simulink model "MCHP_SMO_MCLV48V300W_dsPIC33CK64MC105_DIM"  (R2022b)
settings: Solver=FixedStepDiscrete  StartTime=0.0  StopTime=10.0  FixedStep=50e-6  RelTol=1e-3  EnableMultiTasking=on
undefined symbols (not defined in the file): A4, B0, C12, C13, C4, C5, C6, C8, C9, DiscIntNeverNeededParam, inverter, Iq_Ref_openLoop, Max, MaxPer, ms, NumBits1, NumBits2, P20, P32, P52, P53, P54, P56, P57, P60, P61, PI_params, Pin, pmsm, PU_System, PWM1max, PWM_frequency, Resol, s, Speed_Ref_openLoop, Ts, Ts_speed, us
libraries: simulink x30, MCHP_Blockset x18, mcbcontrolslib x9, slpidlib x3, mcbplantlib x1, autolibpmsmexterior x1
(part 3 of 4)

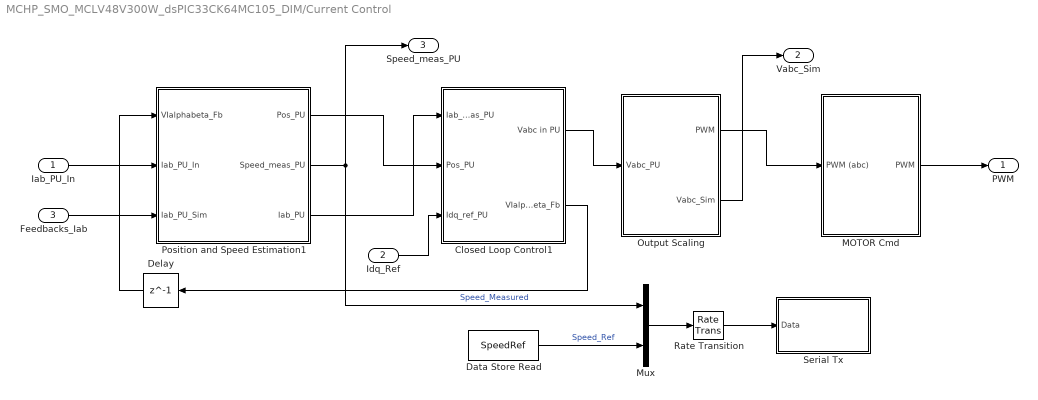
== system MCHP_SMO_MCLV48V300W_dsPIC33CK64MC105_DIM/Current Control ==
  Iab_PU_In : Inport
  Idq_Ref : Inport  Port=2
  Feedbacks_Iab : Inport  Port=3
  Closed Loop Control1 : Subsystem
  Data Store Read : DataStoreRead  DataStoreName=SpeedRef  IndexOptions=Index vector (dialog)  Indices=1  OutputSizes=1
  Delay : Delay  DelayLength=1
  MOTOR Cmd : Subsystem
  Mux : Mux  Inputs=2
  Output Scaling : Subsystem
  Position and Speed Estimation1 : Subsystem
  Rate Transition : RateTransition  Integrity=off  Deterministic=off  OutPortSampleTime=Ts*100
  Serial Tx : Subsystem
  PWM : Outport
  Vabc_Sim : Outport  Port=2
  Speed_meas_PU : Outport  Port=3
  wires:
  Output Scaling/1(PWM) -> MOTOR Cmd/1(PWM (abc))
  Closed Loop Control1/1(Vabc in PU) -> Output Scaling/1(Vabc_PU)
  MOTOR Cmd/1(PWM) -> PWM/1
  Iab_PU_In/1 -> Position and Speed Estimation1/2(Iab_PU_In)
  Closed Loop Control1/2(VIalphabeta_Fb) -> Delay/1
  Delay/1 -> Position and Speed Estimation1/1(VIalphabeta_Fb)
  Idq_Ref/1 -> Closed Loop Control1/3(Idq_ref_PU)
  Position and Speed Estimation1/1(Pos_PU) -> Closed Loop Control1/2(Pos_PU)
  Position and Speed Estimation1/3(Iab_PU) -> Closed Loop Control1/1(Iab_meas_PU)
  Feedbacks_Iab/1 -> Position and Speed Estimation1/3(Iab_PU_Sim)
  Output Scaling/2(Vabc_Sim) -> Vabc_Sim/1
  Data Store Read/1 -> Mux/2  "Speed_Ref"
  Rate Transition/1 -> Serial Tx/1(Data)
  Position and Speed Estimation1/2(Speed_meas_PU) -> Mux/1, Speed_meas_PU/1  "Speed_Measured"
  Mux/1 -> Rate Transition/1

== system MCHP_SMO_MCLV48V300W_dsPIC33CK64MC105_DIM/Inverter and Motor ==
  Duty_Cycles : Inport
  Codegeneration : Subsystem
  Simulation : Subsystem
  Variant Sink : VariantSink
  Variant Source : VariantSource
  Feedbacks_Iab : Outport  VectorParamsAs1DForOutWhenUnconnected=off
  wires:
  Codegeneration/1(Feedbacks_Iab) -> Variant Source/1
  Variant Sink/1 -> Codegeneration/1(Duty_Cycles)
  Simulation/1(Feedbacks_Iab) -> Variant Source/2
  Variant Sink/2 -> Simulation/1(Duty_Cycles)
  Variant Source/1 -> Feedbacks_Iab/1
  Duty_Cycles/1 -> Variant Sink/1

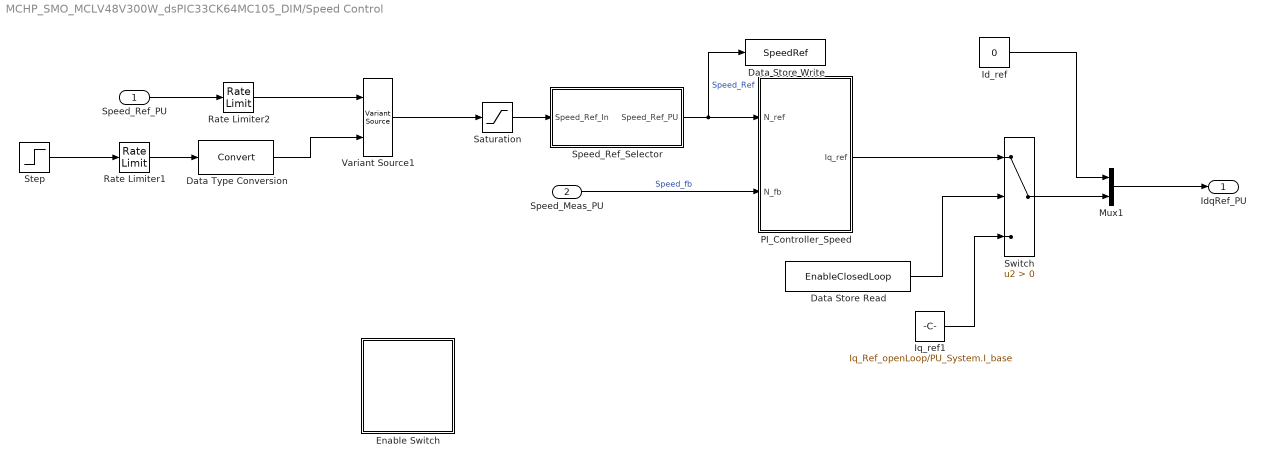
== system MCHP_SMO_MCLV48V300W_dsPIC33CK64MC105_DIM/Speed Control ==
  Speed_Ref_PU : Inport
  Speed_Meas_PU : Inport  Port=2
  Data Store Read : DataStoreRead  DataStoreName=EnableClosedLoop  IndexOptions=Index vector (dialog)  Indices=1  OutputSizes=1
  Data Store Write : DataStoreWrite  DataStoreName=SpeedRef  IndexOptions=Index vector (dialog)  Indices=1  OutputSizes=1
  Data Type Conversion : DataTypeConversion  SaturateOnIntegerOverflow=off  RndMeth=Floor
  Enable Switch : Subsystem  Variant=on  VariantControlMode=sim codegen switching
  Id_ref : Constant  Value=0  OutDataTypeStr=dataType  SampleTime=Ts_speed
  Iq_ref1 : Constant  Value=Iq_Ref_openLoop/PU_System.I_base  OutDataTypeStr=dataType  SampleTime=Ts_speed
  Mux1 : Mux  Inputs=2
  PI_Controller_Speed : Subsystem
  Rate Limiter1 : RateLimiter  RisingSlewLimit=0.5  FallingSlewLimit=-0.2  SampleTimeMode=inherited
  Rate Limiter2 : RateLimiter  RisingSlewLimit=0.5  FallingSlewLimit=-0.2  SampleTimeMode=inherited
  Saturation : Saturate  UpperLimit=(pmsm.N_max/PU_System.N_base)  LowerLimit=Speed_Ref_openLoop/PU_System.N_base
  Speed_Ref_Selector : Subsystem
  Step : Step  Time=5.5  Before=Speed_Ref_openLoop/PU_System.N_base
  Switch : Switch  Criteria=u2 > Threshold  SaturateOnIntegerOverflow=off  InputSameDT=off
  Variant Source1 : VariantSource
  IdqRef_PU : Outport  VectorParamsAs1DForOutWhenUnconnected=off
  wires:
  PI_Controller_Speed/1(Iq_ref) -> Switch/1
  Saturation/1 -> Speed_Ref_Selector/1(Speed_Ref_In)
  Data Store Read/1 -> Switch/2
  Iq_ref1/1 -> Switch/3
  Mux1/1 -> IdqRef_PU/1
  Speed_Ref_PU/1 -> Rate Limiter2/1
  Switch/1 -> Mux1/2
  Speed_Ref_Selector/1(Speed_Ref_PU) -> Data Store Write/1, PI_Controller_Speed/1(N_ref)  "Speed_Ref"
  Id_ref/1 -> Mux1/1
  Speed_Meas_PU/1 -> PI_Controller_Speed/2(N_fb)  "Speed_fb"
  Rate Limiter1/1 -> Data Type Conversion/1
  Data Type Conversion/1 -> Variant Source1/2
  Step/1 -> Rate Limiter1/1
  Rate Limiter2/1 -> Variant Source1/1
  Variant Source1/1 -> Saturation/1

== system MCHP_SMO_MCLV48V300W_dsPIC33CK64MC105_DIM/Triggered Subsystem ==
  Trigger : TriggerPort  TriggerType=falling  VariantControl=Variant
  Data Store Write : DataStoreWrite  DataStoreName=Enable  IndexOptions=Index vector (dialog)  Indices=1  OutputSizes=1
  Delay : Delay  DelayLength=1  InitialCondition=0
  NOT : Logic  Operator=NOT  IconShape=distinctive  AllPortsSameDT=off  OutDataTypeStr=boolean
  wires:
  NOT/1 -> Data Store Write/1, Delay/1
  Delay/1 -> NOT/1

== system MCHP_SMO_MCLV48V300W_dsPIC33CK64MC105_DIM/BOARD MCLV-48V-300W dsPIC33CK64MC105 MC DIM/ADC ==
  ADC dsPIC High Speed SAR Motor Currents : MCHP_Blockset/Analog IO/ADC dsPIC High Speed SAR  ACLKCON=Optimized for PWM resolution & ADC conversion speed  ADC_FRACT=Fractional (left aligned)  ADC_NRE=off  DMA_Size=Single trigger - (default)  ADC_Synchronisation=Triggered by custom source  ADC_Trig=Dynamic Options  ADC_Trig_TXT=PWM1 Trigger 1  ADC_TrigTimeStep=Trig model step after all sample from this block are converted  ADC_TrigInfo=0  SampleTime=50e-6  S_INPUT=[]  S_INPUT_Size=[]  S_OUTPUT="[5  5]"  S_OUTPUT_Size="[1  1]"  S_ListCustomDatatype=S.S_ListCustomDatatype={};  MCHP_USER_INTERRUPTS={ADCAN-1}{ADCBUF-1}{ADC Data -1 Ready}{VectorName(ADCAN-1Interrupt) Priority(-1) RegisterReadClear(ADCBUF-1)Config_BitSet(ADIELbits.IE-1) };{ADCAN0}{ADCBUF0}{ADC Data 0 Ready}{VectorName(ADCAN0Interrupt) Priority(-1) RegisterReadClear(ADCBUF0)Config_BitSet(ADIELbits.IE0) };  MCHP_PORT={Analog Input 0}{AN0}15:2:A0;{Analog Input 1}{AN1}15:2:B2;  MCHP_MASTERLINK=MCHP_SMO_MCLV48V300W_dsPIC33CK64MC105_DIM/BOARD MCLV-48V-300W dsPIC33CK64MC105 MC DIM/Microchip Master  MCHP_CRC=3793139  ADC_Info=Total Time = 1.32(us)  ADC0_pin=Dynamic Options  ADC0_pin_TXT=Not used  ADC0_R="< 5    kOhm"  ADC0_res=12 bits  ADC0_signed=signed 16 bits  ADC0_FILTER=No Oversampling  ADC0_FILTER_nSamples=256 samples  ADC0_STRGEN=End sampling and start conversion  ADC0_STRGEN_on=Start sampling followed by conversion  ADC0_SSAMPEN=off  ADC0_Info=tSmp_min=20(ns) x 0 = 0(s) ; tConv=210(ns) x 0 = 0(s) ; TOTAL=0(s)  ADC1_pin=Dynamic Options  ADC1_pin_TXT=Not used  ADC1_R="< 5    kOhm"  ADC1_res=12 bits  ADC1_signed=signed 16 bits  ADC1_FILTER=No Oversampling  ADC1_FILTER_nSamples=128 samples  ADC1_STRGEN=End sampling and start conversion  ADC1_STRGEN_on=Start sampling followed by conversion  ADC1_SSAMPEN=off  ADC1_Info=tSmp_min=260(ns) x 0 = 0(s) ; tConv=370(ns) x 1 = 370(ns) ; TOTAL=380(ns)  ADC2_pin=Dynamic Options  ADC2_pin_TXT=Not used  ADC2_R="< 5    kOhm"  ADC2_res=12 bits  ADC2_signed=signed 16 bits  ADC2_FILTER=No Oversampling  ADC2_FILTER_nSamples=256 samples  ADC2_STRGEN=End sampling and start conversion  ADC2_STRGEN_on=Start sampling followed by conversion  ADC2_SSAMPEN=on  ADC2_Info=tSmp_min=14.706(ns) x 0 = 0(s) ; tConv=154.41(ns) x 0 = 0(s) ; TOTAL=0(s)  ADC3_pin=Dynamic Options  ADC3_pin_TXT=Not used  ADC3_R="< 10   kOhm"  ADC3_res=12 bits  ADC3_signed=signed 16 bits  ADC3_FILTER=Burst convert of n samples are Summed  ADC3_FILTER_nSamples=64 samples  ADC3_STRGEN=End sampling and start conversion  ADC3_STRGEN_on=Start sampling followed by conversion  ADC3_SSAMPEN=on  ADC3_Info=tSmp_min=14.706(ns) x 0 = 0(s) ; tConv=154.41(ns) x 0 = 0(s) ; TOTAL=0(s)  ADC4_pin=Dynamic Options  ADC4_pin_TXT=Not used  ADC4_R=< 200 Ohm  ADC4_res=12 bits  ADC4_signed=unsigned 16 bits  ADC4_FILTER=No Oversampling  ADC4_FILTER_nSamples=256 samples  ADC4_STRGEN=End sampling and start conversion  ADC4_STRGEN_on=Start sampling followed by conversion  ADC4_SSAMPEN=off  ADC4_Info=tSmp_min=14.706(ns) x 0 = 0(s) ; tConv=154.41(ns) x 0 = 0(s) ; TOTAL=0(s)  ADC5_pin=Dynamic Options  ADC5_pin_TXT=Not used  ADC5_R=< 200 Ohm  ADC5_res=12 bits  ADC5_signed=unsigned 16 bits  ADC5_FILTER=Burst convert of n samples are Summed  ADC5_FILTER_nSamples=256 samples  ADC5_STRGEN=End sampling and start conversion  ADC5_STRGEN_on=Start sampling followed by conversion  ADC5_SSAMPEN=on  ADC5_Info=tSmp_min=14.706(ns) x 0 = 0(s) ; tConv=154.41(ns) x 0 = 0(s) ; TOTAL=0(s)  ADC6_pin=Dynamic Options  ADC6_pin_TXT=Not used  ADC6_R=< 200 Ohm  ADC6_res=12 bits  ADC6_signed=unsigned 16 bits  ADC6_FILTER=Burst convert of n samples are Summed  ADC6_FILTER_nSamples=256 samples  ADC6_STRGEN=End sampling and start conversion  ADC6_STRGEN_on=Start sampling followed by conversion  ADC6_SSAMPEN=on  ADC6_Info=tSmp_min=14.706(ns) x 0 = 0(s) ; tConv=154.41(ns) x 0 = 0(s) ; TOTAL=0(s)  ADC7_R="< 5    kOhm"  ADC7_res=12 bits  ADC7_AN0=signed int16  ADC7_AN1=signed int16  ADC7_AN2=Not used  ADC7_AN3=Not used  ADC7_AN4=Not used  ADC7_AN5=Not used  ADC7_AN6=Not used  ADC7_AN7=Not used  ADC7_AN8=Not used  ADC7_AN9=Not used  ADC7_AN10=Not used  ADC7_AN11=Not used  ADC7_AN12=Not used  ADC7_AN13=Not used  ADC7_AN14=Not used  ADC7_AN15=Not used  ADC7_AN16=Not used  ADC7_AN17=Not used  ADC7_AN18=Not used  ADC7_AN19=Not used  ADC7_AN20=Not used  ADC7_AN21=Not used  ADC7_AN22=Not used  ADC7_AN23=Not used  ADC7_AN24=Not used  ADC7_AN25=Not used  ADC7_AN26=Not used  ADC7_AN27=Not used  ADC7_AN28=Not used  ADC7_AN29=Not used  ADC7_AN30=Not used  ADC7_AN31=Not used  IVref=Not used  IVTemp=Not used  ADC7_Info=tSmp_min=280(ns) x 2 = 560(ns) ; tConv=370(ns) x 2 = 740(ns) ; TOTAL=1.32(us)
      settings: SourceProductName=MPLAB Device Blocks for Simulink
  ADC dsPIC High Speed SAR others : MCHP_Blockset/Analog IO/ADC dsPIC High Speed SAR  ACLKCON=Not used  ADC_FRACT=Fractional (left aligned)  ADC_NRE=off  DMA_Size=Single trigger - (default)  ADC_Synchronisation=Triggered by custom source  ADC_Trig=Dynamic Options  ADC_Trig_TXT=PWM1 Trigger 1  ADC_TrigTimeStep=None (independant)  ADC_TrigInfo=0  SampleTime=50e-6  S_INPUT=[]  S_INPUT_Size=[]  S_OUTPUT="[5  5]"  S_OUTPUT_Size="[1  1]"  S_ListCustomDatatype=S.S_ListCustomDatatype={};  MCHP_USER_INTERRUPTS={ADCAN3}{ADCBUF3}{ADC Data 3 Ready}{VectorName(ADCAN3Interrupt) Priority(-1) RegisterReadClear(ADCBUF3)Config_BitSet(ADIELbits.IE3) };{ADCAN9}{ADCBUF9}{ADC Data 9 Ready}{VectorName(ADCAN9Interrupt) Priority(-1) RegisterReadClear(ADCBUF9)Config_BitSet(ADIELbits.IE9) };{ADCAN10}{ADCBUF10}{ADC Data 10 Ready}{VectorName(ADCAN10Interrupt) Priority(-1) RegisterReadClear(ADCBUF10)Config_BitSet(ADIELbits.IE10) };  MCHP_PORT={Analog Input 4}{AN4}15:2:A4;{Analog Input 10}{AN10}15:2:B8;{Analog Input 11}{AN11}15:2:B9;  MCHP_MASTERLINK=MCHP_SMO_MCLV48V300W_dsPIC33CK64MC105_DIM/BOARD MCLV-48V-300W dsPIC33CK64MC105 MC DIM/Microchip Master  MCHP_CRC=3894852  ADC_Info=Total Time = 1.98(us)  ADC0_pin=Dynamic Options  ADC0_pin_TXT=Not used  ADC0_R="< 5    kOhm"  ADC0_res=12 bits  ADC0_signed=signed 16 bits  ADC0_FILTER=No Oversampling  ADC0_FILTER_nSamples=256 samples  ADC0_STRGEN=Start sampling followed by conversion  ADC0_STRGEN_on=Start sampling followed by conversion  ADC0_SSAMPEN=off  ADC0_Info=tSmp_min=260(ns) x 1 = 260(ns) ; tConv=370(ns) x 1 = 370(ns) ; TOTAL=640(ns)  ADC1_pin=Dynamic Options  ADC1_pin_TXT=Not used  ADC1_R="< 5    kOhm"  ADC1_res=12 bits  ADC1_signed=signed 16 bits  ADC1_FILTER=No Oversampling  ADC1_FILTER_nSamples=128 samples  ADC1_STRGEN=Start sampling followed by conversion  ADC1_STRGEN_on=Start sampling followed by conversion  ADC1_SSAMPEN=off  ADC1_Info=tSmp_min=20(ns) x 0 = 0(s) ; tConv=210(ns) x 0 = 0(s) ; TOTAL=0(s)  ADC2_pin=Dynamic Options  ADC2_pin_TXT=Not used  ADC2_R="< 5    kOhm"  ADC2_res=12 bits  ADC2_signed=signed 16 bits  ADC2_FILTER=No Oversampling  ADC2_FILTER_nSamples=256 samples  ADC2_STRGEN=End sampling and start conversion  ADC2_STRGEN_on=Start sampling followed by conversion  ADC2_SSAMPEN=on  ADC2_Info=tSmp_min=14.706(ns) x 0 = 0(s) ; tConv=154.41(ns) x 0 = 0(s) ; TOTAL=0(s)  ADC3_pin=Dynamic Options  ADC3_pin_TXT=Not used  ADC3_R="< 10   kOhm"  ADC3_res=12 bits  ADC3_signed=signed 16 bits  ADC3_FILTER=Burst convert of n samples are Summed  ADC3_FILTER_nSamples=64 samples  ADC3_STRGEN=End sampling and start conversion  ADC3_STRGEN_on=Start sampling followed by conversion  ADC3_SSAMPEN=on  ADC3_Info=tSmp_min=14.706(ns) x 0 = 0(s) ; tConv=154.41(ns) x 0 = 0(s) ; TOTAL=0(s)  ADC4_pin=Dynamic Options  ADC4_pin_TXT=Not used  ADC4_R=< 200 Ohm  ADC4_res=12 bits  ADC4_signed=unsigned 16 bits  ADC4_FILTER=No Oversampling  ADC4_FILTER_nSamples=256 samples  ADC4_STRGEN=End sampling and start conversion  ADC4_STRGEN_on=Start sampling followed by conversion  ADC4_SSAMPEN=off  ADC4_Info=tSmp_min=14.706(ns) x 0 = 0(s) ; tConv=154.41(ns) x 0 = 0(s) ; TOTAL=0(s)  ADC5_pin=Dynamic Options  ADC5_pin_TXT=Not used  ADC5_R=< 200 Ohm  ADC5_res=12 bits  ADC5_signed=unsigned 16 bits  ADC5_FILTER=Burst convert of n samples are Summed  ADC5_FILTER_nSamples=256 samples  ADC5_STRGEN=End sampling and start conversion  ADC5_STRGEN_on=Start sampling followed by conversion  ADC5_SSAMPEN=on  ADC5_Info=tSmp_min=14.706(ns) x 0 = 0(s) ; tConv=154.41(ns) x 0 = 0(s) ; TOTAL=0(s)  ADC6_pin=Dynamic Options  ADC6_pin_TXT=Not used  ADC6_R=< 200 Ohm  ADC6_res=12 bits  ADC6_signed=unsigned 16 bits  ADC6_FILTER=Burst convert of n samples are Summed  ADC6_FILTER_nSamples=256 samples  ADC6_STRGEN=End sampling and start conversion  ADC6_STRGEN_on=Start sampling followed by conversion  ADC6_SSAMPEN=on  ADC6_Info=tSmp_min=14.706(ns) x 0 = 0(s) ; tConv=154.41(ns) x 0 = 0(s) ; TOTAL=0(s)  ADC7_R="< 5    kOhm"  ADC7_res=12 bits  ADC7_AN0=Not used  ADC7_AN1=Not used  ADC7_AN2=Not used  ADC7_AN3=Not used  ADC7_AN4=signed int16  ADC7_AN5=Not used  ADC7_AN6=Not used  ADC7_AN7=Not used  ADC7_AN8=Not used  ADC7_AN9=Not used  ADC7_AN10=unsigned int16  ADC7_AN11=unsigned int16  ADC7_AN12=Not used  ADC7_AN13=Not used  ADC7_AN14=Not used  ADC7_AN15=Not used  ADC7_AN16=Not used  ADC7_AN17=Not used  ADC7_AN18=Not used  ADC7_AN19=Not used  ADC7_AN20=Not used  ADC7_AN21=Not used  ADC7_AN22=Not used  ADC7_AN23=Not used  ADC7_AN24=Not used  ADC7_AN25=Not used  ADC7_AN26=Not used  ADC7_AN27=Not used  ADC7_AN28=Not used  ADC7_AN29=Not used  ADC7_AN30=Not used  ADC7_AN31=Not used  IVref=Not used  IVTemp=Not used  ADC7_Info=tSmp_min=280(ns) x 3 = 840(ns) ; tConv=370(ns) x 3 = 1.11(us) ; TOTAL=1.98(us)
      settings: SourceProductName=MPLAB Device Blocks for Simulink
  Ia : Outport  VectorParamsAs1DForOutWhenUnconnected=off
  Ib : Outport  Port=2  VectorParamsAs1DForOutWhenUnconnected=off
  IBus : Outport  Port=3  VectorParamsAs1DForOutWhenUnconnected=off
  pot : Outport  Port=4  VectorParamsAs1DForOutWhenUnconnected=off
  V_BUS : Outport  Port=5  VectorParamsAs1DForOutWhenUnconnected=off
  wires:
  ADC dsPIC High Speed SAR others/3 -> pot/1
  ADC dsPIC High Speed SAR others/2 -> V_BUS/1
  ADC dsPIC High Speed SAR Motor Currents/1 -> Ia/1
  ADC dsPIC High Speed SAR Motor Currents/2 -> Ib/1
  ADC dsPIC High Speed SAR others/1 -> IBus/1

== system MCHP_SMO_MCLV48V300W_dsPIC33CK64MC105_DIM/BOARD MCLV-48V-300W dsPIC33CK64MC105 MC DIM/Center & sign reversal ==
  I_ab : Inport
  Bias Update : Inport  Port=2
  Average and Sign reverse : Sum  Inputs=+-  SaturateOnIntegerOverflow=on  OutDataTypeStr=Inherit: Same as first input
  Downsample Averaged 2000 samples remove bias : Subsystem  mask{DownSample=2000}
      mask prompts: DownSample "DownSample Factor"
  Rate Transition1 : RateTransition  Deterministic=off
  Iab : Outport
  wires:
  I_ab/1 -> Average and Sign reverse/2, Downsample Averaged 2000 samples remove bias/1(In1)
  Bias Update/1 -> Downsample Averaged 2000 samples remove bias/Enable
  Downsample Averaged 2000 samples remove bias/1(Out1) -> Rate Transition1/1
  Rate Transition1/1 -> Average and Sign reverse/1
  Average and Sign reverse/1 -> Iab/1  "I_ab_raw"

== system MCHP_SMO_MCLV48V300W_dsPIC33CK64MC105_DIM/BOARD MCLV-48V-300W dsPIC33CK64MC105 MC DIM/Downsample Averaged x20 ==
  note: DownSample & Average by changing data scaling
  In1 : Inport
  Compare To Constant : simulink/Logic and Bit Operations/Compare To Constant  relop===  const=1  OutDataTypeStr=boolean
  Counter Limited : simulink/Sources/Counter Limited  uplimit=DownSample-1  tsamp=-1
  Data Type Duplicate : DataTypeDuplicate
  Data Type Propagation : simulink/Signal Attributes/Data Type Propagation  PropDataType=fixdt(1, 16)  IfRefDouble=double  IfRefSingle=single  IsSigned=IsSigned1 or IsSigned2  NumBitsBase=NumBits1+NumBits2  NumBitsMult=1  NumBitsAdd=0  NumBitsAllowFinal=1:128  PropScaling=2^-10  ValuesUsedBestPrec=[5 -7]  SlopeBase=Slope1  SlopeMult=1  SlopeAdd=0  BiasBase=Bias1  BiasMult=1  BiasAdd=0
  Data Type Propagation1 : simulink/Signal Attributes/Data Type Propagation  PropDataType=fixdt(1, 16)  IfRefDouble=double  IfRefSingle=single  IsSigned=IsSigned1 or IsSigned2  NumBitsBase=NumBits1+NumBits2  NumBitsMult=1  NumBitsAdd=0  NumBitsAllowFinal=1:128  PropScaling=2^-10  ValuesUsedBestPrec=[5 -7]  SlopeBase=PosRange1  SlopeMult=1  SlopeAdd=0  BiasBase=Bias1  BiasMult=1  BiasAdd=0
  Discrete-Time Integrator : DiscreteIntegrator  IntegratorMethod=Accumulation: Backward Euler  gainval=1  ExternalReset=sampled level  SampleTime=-1  OutDataTypeStr=Inherit: Inherit via back propagation  ICPrevOutput=DiscIntNeverNeededParam  ICPrevScaledInput=DiscIntNeverNeededParam
  Gain : Gain  Gain=1/DownSample  OutDataTypeStr=Inherit: Inherit via back propagation  RndMeth=Round
  Gain1 : Gain  Gain=1/DownSample  OutDataTypeStr=Inherit: Inherit via back propagation
  Rate Transition1 : RateTransition  OutPortSampleTimeOpt=Multiple of input port sample time  OutPortSampleTimeMultiple=DownSample  OutPortSampleTime=DownSample
  Rate Transition3 : RateTransition  OutPortSampleTimeOpt=Multiple of input port sample time  OutPortSampleTimeMultiple=DownSample  OutPortSampleTime=DownSample
  Terminator : Terminator
  Out1 : Outport  VectorParamsAs1DForOutWhenUnconnected=off
  wires:
  Gain1/1 -> Data Type Propagation1/3, Terminator/1
  Rate Transition1/1 -> Data Type Duplicate/1, Data Type Propagation1/1, Data Type Propagation1/2
  Gain/1 -> Out1/1, Data Type Duplicate/2
  Counter Limited/1 -> Compare To Constant/1
  Discrete-Time Integrator/1 -> Rate Transition3/1, Data Type Propagation/3
  Compare To Constant/1 -> Discrete-Time Integrator/2
  In1/1 -> Data Type Propagation/1, Data Type Propagation/2, Discrete-Time Integrator/1, Rate Transition1/1
  Rate Transition3/1 -> Gain/1, Gain1/1

== system MCHP_SMO_MCLV48V300W_dsPIC33CK64MC105_DIM/BOARD MCLV-48V-300W dsPIC33CK64MC105 MC DIM/Downsample x20 ==
  note: DownSample & Average by changing data scaling
  In1 : Inport
  Compare To Constant : simulink/Logic and Bit Operations/Compare To Constant  relop===  const=1  OutDataTypeStr=boolean
  Counter Limited : simulink/Sources/Counter Limited  uplimit=DownSample-1  tsamp=-1
  Data Type Duplicate : DataTypeDuplicate
  Data Type Propagation : simulink/Signal Attributes/Data Type Propagation  PropDataType=fixdt(1, 16)  IfRefDouble=double  IfRefSingle=single  IsSigned=IsSigned1 or IsSigned2  NumBitsBase=NumBits1+NumBits2  NumBitsMult=1  NumBitsAdd=0  NumBitsAllowFinal=1:128  PropScaling=2^-10  ValuesUsedBestPrec=[5 -7]  SlopeBase=Slope1  SlopeMult=1  SlopeAdd=0  BiasBase=Bias1  BiasMult=1  BiasAdd=0
  Data Type Propagation1 : simulink/Signal Attributes/Data Type Propagation  PropDataType=fixdt(1, 16)  IfRefDouble=double  IfRefSingle=single  IsSigned=IsSigned1 or IsSigned2  NumBitsBase=NumBits1+NumBits2  NumBitsMult=1  NumBitsAdd=0  NumBitsAllowFinal=1:128  PropScaling=2^-10  ValuesUsedBestPrec=[5 -7]  SlopeBase=PosRange1  SlopeMult=1  SlopeAdd=0  BiasBase=Bias1  BiasMult=1  BiasAdd=0
  Discrete-Time Integrator : DiscreteIntegrator  IntegratorMethod=Accumulation: Backward Euler  gainval=1  ExternalReset=sampled level  SampleTime=-1  OutDataTypeStr=Inherit: Inherit via back propagation  ICPrevOutput=DiscIntNeverNeededParam  ICPrevScaledInput=DiscIntNeverNeededParam
  Gain : Gain  Gain=1/DownSample  OutDataTypeStr=Inherit: Inherit via back propagation  RndMeth=Round
  Gain1 : Gain  Gain=1/DownSample  OutDataTypeStr=Inherit: Inherit via back propagation
  Rate Transition1 : RateTransition  OutPortSampleTimeOpt=Multiple of input port sample time  OutPortSampleTimeMultiple=DownSample  OutPortSampleTime=DownSample
  Rate Transition3 : RateTransition  OutPortSampleTimeOpt=Multiple of input port sample time  OutPortSampleTimeMultiple=DownSample  OutPortSampleTime=DownSample
  Terminator : Terminator
  Out1 : Outport  VectorParamsAs1DForOutWhenUnconnected=off
  wires:
  Rate Transition3/1 -> Gain1/1, Gain/1
  In1/1 -> Rate Transition1/1, Discrete-Time Integrator/1, Data Type Propagation/2, Data Type Propagation/1
  Compare To Constant/1 -> Discrete-Time Integrator/2
  Discrete-Time Integrator/1 -> Data Type Propagation/3, Rate Transition3/1
  Counter Limited/1 -> Compare To Constant/1
  Gain/1 -> Data Type Duplicate/2, Out1/1
  Rate Transition1/1 -> Data Type Propagation1/2, Data Type Propagation1/1, Data Type Duplicate/1
  Gain1/1 -> Terminator/1, Data Type Propagation1/3

== system MCHP_SMO_MCLV48V300W_dsPIC33CK64MC105_DIM/BOARD MCLV-48V-300W dsPIC33CK64MC105 MC DIM/Downsample x20 _ ==
  note: DownSample & Average by changing data scaling
  In1 : Inport
  Compare To Constant : simulink/Logic and Bit Operations/Compare To Constant  relop===  const=1  OutDataTypeStr=boolean
  Counter Limited : simulink/Sources/Counter Limited  uplimit=DownSample-1  tsamp=-1
  Data Type Duplicate : DataTypeDuplicate
  Data Type Propagation : simulink/Signal Attributes/Data Type Propagation  PropDataType=fixdt(1, 16)  IfRefDouble=double  IfRefSingle=single  IsSigned=IsSigned1 or IsSigned2  NumBitsBase=NumBits1+NumBits2  NumBitsMult=1  NumBitsAdd=0  NumBitsAllowFinal=1:128  PropScaling=2^-10  ValuesUsedBestPrec=[5 -7]  SlopeBase=Slope1  SlopeMult=1  SlopeAdd=0  BiasBase=Bias1  BiasMult=1  BiasAdd=0
  Data Type Propagation1 : simulink/Signal Attributes/Data Type Propagation  PropDataType=fixdt(1, 16)  IfRefDouble=double  IfRefSingle=single  IsSigned=IsSigned1 or IsSigned2  NumBitsBase=NumBits1+NumBits2  NumBitsMult=1  NumBitsAdd=0  NumBitsAllowFinal=1:128  PropScaling=2^-10  ValuesUsedBestPrec=[5 -7]  SlopeBase=PosRange1  SlopeMult=1  SlopeAdd=0  BiasBase=Bias1  BiasMult=1  BiasAdd=0
  Discrete-Time Integrator : DiscreteIntegrator  IntegratorMethod=Accumulation: Backward Euler  gainval=1  ExternalReset=sampled level  SampleTime=-1  OutDataTypeStr=Inherit: Inherit via back propagation  ICPrevOutput=DiscIntNeverNeededParam  ICPrevScaledInput=DiscIntNeverNeededParam
  Gain : Gain  Gain=1/DownSample  OutDataTypeStr=Inherit: Inherit via back propagation  RndMeth=Round
  Gain1 : Gain  Gain=1/DownSample  OutDataTypeStr=Inherit: Inherit via back propagation
  Rate Transition1 : RateTransition  OutPortSampleTimeOpt=Multiple of input port sample time  OutPortSampleTimeMultiple=DownSample  OutPortSampleTime=DownSample
  Rate Transition3 : RateTransition  OutPortSampleTimeOpt=Multiple of input port sample time  OutPortSampleTimeMultiple=DownSample  OutPortSampleTime=DownSample
  Terminator : Terminator
  Out1 : Outport  VectorParamsAs1DForOutWhenUnconnected=off
  wires:
  Gain1/1 -> Data Type Propagation1/3, Terminator/1
  Rate Transition1/1 -> Data Type Duplicate/1, Data Type Propagation1/1, Data Type Propagation1/2
  Gain/1 -> Out1/1, Data Type Duplicate/2
  Counter Limited/1 -> Compare To Constant/1
  Discrete-Time Integrator/1 -> Rate Transition3/1, Data Type Propagation/3
  Compare To Constant/1 -> Discrete-Time Integrator/2
  In1/1 -> Data Type Propagation/1, Data Type Propagation/2, Discrete-Time Integrator/1, Rate Transition1/1
  Rate Transition3/1 -> Gain/1, Gain1/1

== system MCHP_SMO_MCLV48V300W_dsPIC33CK64MC105_DIM/BOARD MCLV-48V-300W dsPIC33CK64MC105 MC DIM/LVMC board webpage ==

== system MCHP_SMO_MCLV48V300W_dsPIC33CK64MC105_DIM/BOARD MCLV-48V-300W dsPIC33CK64MC105 MC DIM/PWM Scaling ==
  vabc [0 1] : Inport
  Gain : Gain  Gain=PWM1max  OutDataTypeStr=uint16
  PWM : Outport  VectorParamsAs1DForOutWhenUnconnected=off
  wires:
  vabc [0 1]/1 -> Gain/1
  Gain/1 -> PWM/1

== system MCHP_SMO_MCLV48V300W_dsPIC33CK64MC105_DIM/BOARD MCLV-48V-300W dsPIC33CK64MC105 MC DIM/Timing Analysis ==
  note: CPU overload is 0 if no overload took place between two MCU Overload block execution.
      | Otherwise, bits field output code for TID(s) responsible for at least one overload.
  Downsample Averaged2 : Subsystem  mask{InputSampleTime=.0005, DownSample=200}
      mask prompts: InputSampleTime "Input sample time"; DownSample "DownSample Factor"
  Gain : Gain  Gain=10e-9/.0005 * 100  OutMin=0  OutMax=100  OutDataTypeStr=fixdt(0,16)  RndMeth=Simplest  SaturateOnIntegerOverflow=on
  MCU Load : MCHP_Blockset/Profiling/MCU Load  MCULoadPin=Dynamic Options  MCULoadPin_TXT=None  MCULoadMeasure=on  TIMER_Resolution=Dynamic Options  TIMER_Resolution_TXT="Resol: 0.01(us)  -  Max: 0.655(ms)"  MCHP_TIMER_REQUEST={MCU_Load}{MCU_Load}21:5:0:0:[]:65536;  MCHP_TIMER_RESULT=[1 65535 ]  MCHP_MASTERLINK=MCHP_SMO_MCLV48V300W_dsPIC33CK64MC105_DIM/BOARD MCLV-48V-300W dsPIC33CK64MC105 MC DIM/Microchip Master  MCHP_COMPILED_INFO="CompiledSampleTime= [0.00050000000000000001041   0 ];CompiledInportDataTypes=[    ];CompiledInportDataWidth=[];"  Info="Timer 1:  Resol: 10(ns)  -  Max: 655.36(us)"  SampleTime=.0005
      settings: SourceProductName=MPLAB Device Blocks for Simulink
  MCU Overload : MCHP_Blockset/Profiling/MCU Overload  MCUOverloadBlockOutput=on  MCUOverLoadPin=Dynamic Options  MCUOverLoadPin_TXT=None  MCHP_MASTERLINK=MCHP_SMO_MCLV48V300W_dsPIC33CK64MC105_DIM/BOARD MCLV-48V-300W dsPIC33CK64MC105 MC DIM/Microchip Master  SampleTime=-1
      settings: SourceProductName=MPLAB Device Blocks for Simulink
  Overload : Constant  Value=65535  OutDataTypeStr=Inherit: Inherit via back propagation
  Rate Transition : RateTransition  Deterministic=off  OutPortSampleTime=.0005*200
  Switch : Switch  Criteria=u2 ~= 0  SaturateOnIntegerOverflow=off  InputSameDT=off
  CPU Load : Outport  Unit=%  SampleTime=.0005*200
  CPU Overload : Outport  Port=2
  wires:
  Rate Transition/1 -> Switch/2
  MCU Overload/1 -> Rate Transition/1, CPU Overload/1
  MCU Load/1 -> Downsample Averaged2/1(In1)
  Downsample Averaged2/1(Out1) -> Switch/3
  Switch/1 -> Gain/1
  Overload/1 -> Switch/1
  Gain/1 -> CPU Load/1

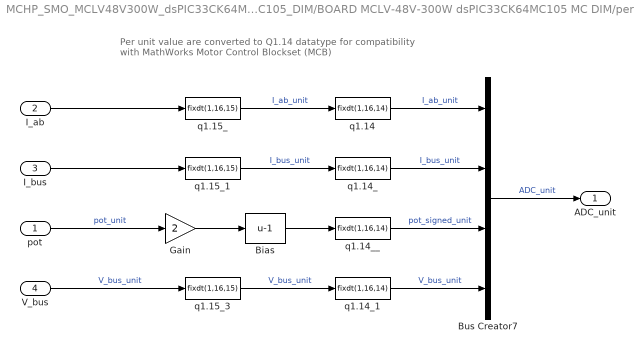
== system MCHP_SMO_MCLV48V300W_dsPIC33CK64MC105_DIM/BOARD MCLV-48V-300W dsPIC33CK64MC105 MC DIM/per_unit ==
  note: Per unit value are converted to Q1.14 datatype
      | for compatibility with MathWorks Motor Control Blockset (MCB)
  pot : Inport
  I_ab : Inport  Port=2
  I_bus : Inport  Port=3
  V_bus : Inport  Port=4
  Bias : Bias  Bias=-1  SaturateOnIntegerOverflow=off
  Bus Creator7 : BusCreator  Inputs=4
  Gain : Gain  Gain=2  OutDataTypeStr=fixdt(1,16,15)  LockScale=on
  q1.14 : DataTypeConversion  OutDataTypeStr=fixdt(1,16,14)  SaturateOnIntegerOverflow=off  RndMeth=Floor  LockScale=on
  q1.14_ : DataTypeConversion  OutDataTypeStr=fixdt(1,16,14)  SaturateOnIntegerOverflow=off  RndMeth=Floor  LockScale=on
  q1.14_1 : DataTypeConversion  OutDataTypeStr=fixdt(1,16,14)  SaturateOnIntegerOverflow=off  RndMeth=Floor  LockScale=on
  q1.14__ : DataTypeConversion  OutDataTypeStr=fixdt(1,16,14)  SaturateOnIntegerOverflow=off  RndMeth=Floor  LockScale=on
  q1.15_ : DataTypeConversion  OutDataTypeStr=fixdt(1,16,15)  ConvertRealWorld=Stored Integer (SI)  SaturateOnIntegerOverflow=off  RndMeth=Floor  LockScale=on
  q1.15_1 : DataTypeConversion  OutDataTypeStr=fixdt(1,16,15)  ConvertRealWorld=Stored Integer (SI)  SaturateOnIntegerOverflow=off  RndMeth=Floor  LockScale=on
  q1.15_3 : DataTypeConversion  OutDataTypeStr=fixdt(1,16,15)  ConvertRealWorld=Stored Integer (SI)  SaturateOnIntegerOverflow=off  RndMeth=Floor  LockScale=on
  ADC_unit : Outport
  wires:
  I_ab/1 -> q1.15_/1
  V_bus/1 -> q1.15_3/1  "V_bus_unit"
  pot/1 -> Gain/1  "pot_unit"
  I_bus/1 -> q1.15_1/1
  q1.15_1/1 -> q1.14_/1  "I_bus_unit"
  q1.15_/1 -> q1.14/1  "I_ab_unit"
  Bus Creator7/1 -> ADC_unit/1  "ADC_unit"
  q1.15_3/1 -> q1.14_1/1  "V_bus_unit"
  q1.14/1 -> Bus Creator7/1  "I_ab_unit"
  q1.14_/1 -> Bus Creator7/2  "I_bus_unit"
  q1.14__/1 -> Bus Creator7/3  "pot_signed_unit"
  q1.14_1/1 -> Bus Creator7/4  "V_bus_unit"
  Gain/1 -> Bias/1
  Bias/1 -> q1.14__/1

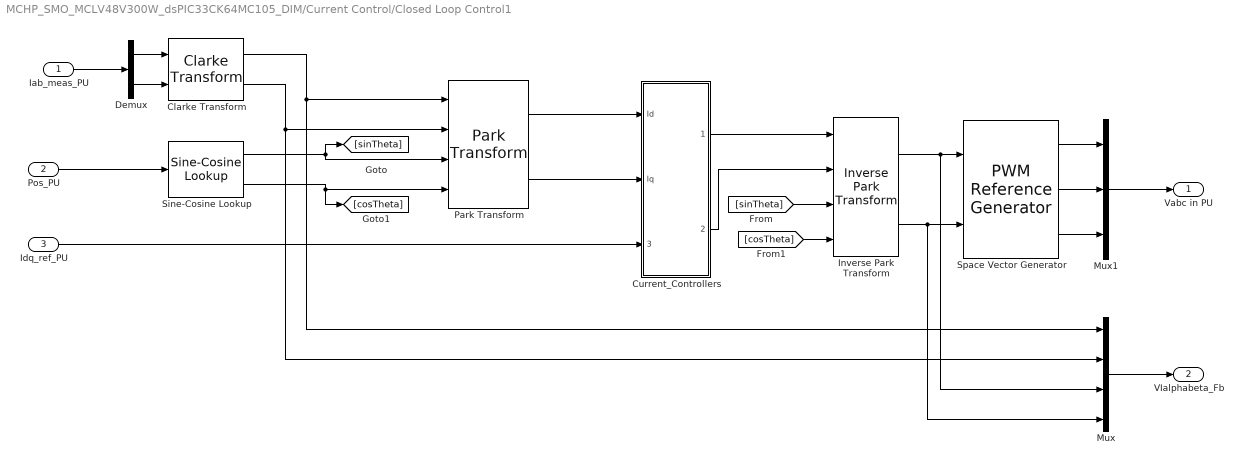
== system MCHP_SMO_MCLV48V300W_dsPIC33CK64MC105_DIM/Current Control/Closed Loop Control1 ==
  Iab_meas_PU : Inport
  Pos_PU : Inport  Port=2
  Idq_ref_PU : Inport  Port=3
  Clarke Transform : mcbcontrolslib/Clarke Transform  VariantControl=Variant2
  Current_Controllers : Subsystem
  Demux : Demux  Outputs=2
  Inverse Park Transform : mcbcontrolslib/Inverse Park Transform  AxisAlignment=D-axis
  Mux : Mux
  Mux1 : Mux  Inputs=3
  Park Transform : mcbcontrolslib/Park Transform  AxisAlignment=D-axis
  Sine-Cosine Lookup : mcbcontrolslib/Sine-Cosine Lookup  AngleInput=Per-unit  N_points=1024
  Space Vector Generator : mcbcontrolslib/PWM Reference Generator  inSignal=Valphabeta  modType=SVM: space vector modulation
  Vabc in PU : Outport  VectorParamsAs1DForOutWhenUnconnected=off
  VIalphabeta_Fb : Outport  Port=2
  wires:
  Current_Controllers/1(Vd_ref) -> Inverse Park Transform/1
  Inverse Park Transform/1 -> Mux/3, Space Vector Generator/1
  Park Transform/1 -> Current_Controllers/1(Id)
  Clarke Transform/1 -> Mux/1, Park Transform/1
  [sinTheta] -> Inverse Park Transform/3
  Sine-Cosine Lookup/1 -> Park Transform/3, [sinTheta]
  Clarke Transform/2 -> Mux/2, Park Transform/2
  Space Vector Generator/1 -> Mux1/1
  Space Vector Generator/3 -> Mux1/3
  Sine-Cosine Lookup/2 -> [cosTheta], Park Transform/4
  Space Vector Generator/2 -> Mux1/2
  Idq_ref_PU/1 -> Current_Controllers/3(Idq_ref_PU)
  Iab_meas_PU/1 -> Demux/1
  Inverse Park Transform/2 -> Mux/4, Space Vector Generator/2
  Demux/1 -> Clarke Transform/1
  Demux/2 -> Clarke Transform/2
  Park Transform/2 -> Current_Controllers/2(Iq)
  [cosTheta] -> Inverse Park Transform/4
  Current_Controllers/2(Vq_ref) -> Inverse Park Transform/2
  Mux1/1 -> Vabc in PU/1
  Pos_PU/1 -> Sine-Cosine Lookup/1
  Mux/1 -> VIalphabeta_Fb/1

== system MCHP_SMO_MCLV48V300W_dsPIC33CK64MC105_DIM/Current Control/MOTOR Cmd ==
  PWM (abc) : Inport
  Dead time Compensation : Bias  Bias=round( (inverter.deadtime/5e-5) )  SaturateOnIntegerOverflow=off
  PWM : Outport
  wires:
  Dead time Compensation/1 -> PWM/1
  PWM (abc)/1 -> Dead time Compensation/1

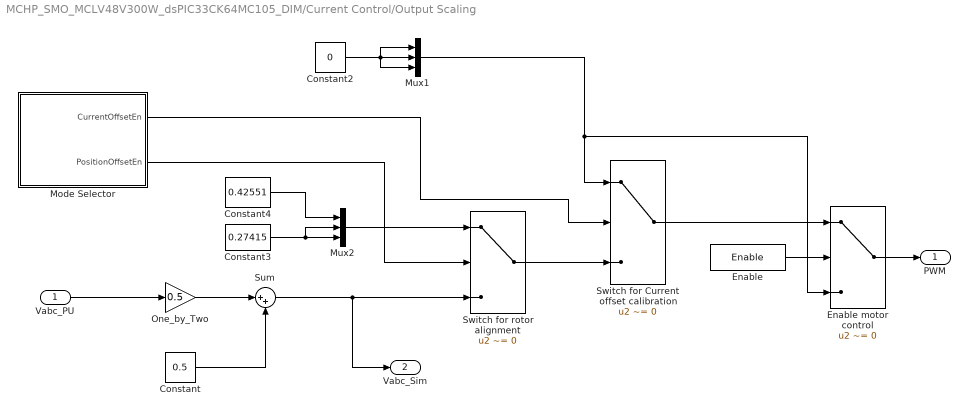
== system MCHP_SMO_MCLV48V300W_dsPIC33CK64MC105_DIM/Current Control/Output Scaling ==
  Vabc_PU : Inport
  Constant : Constant  Value=0.5  OutDataTypeStr=dataType  SampleTime=-1
  Constant2 : Constant  Value=0  OutDataTypeStr=Inherit: Inherit via back propagation
  Constant3 : Constant  Value=0.27415  OutDataTypeStr=Inherit: Inherit via back propagation
  Constant4 : Constant  Value=0.42551  OutDataTypeStr=Inherit: Inherit via back propagation
  Enable : DataStoreRead  DataStoreName=Enable  IndexOptions=Index vector (dialog)  Indices=1  OutputSizes=1
  Enable motor control : Switch  Criteria=u2 ~= 0  Threshold=250  SaturateOnIntegerOverflow=off  InputSameDT=off
  Mode Selector : Subsystem
  Mux1 : Mux  Inputs=3
  Mux2 : Mux  Inputs=3
  One_by_Two : Gain  Gain=0.5  RndMeth=Simplest  OutDataTypeStr=Inherit: Same as input
  Sum : Sum  Inputs=|++
  Switch for Current offset calibration : Switch  Criteria=u2 ~= 0  Threshold=250  SaturateOnIntegerOverflow=off  InputSameDT=off
  Switch for rotor alignment : Switch  Criteria=u2 ~= 0  Threshold=250  SaturateOnIntegerOverflow=off  InputSameDT=off
  PWM : Outport
  Vabc_Sim : Outport  Port=2
  wires:
  Constant/1 -> Sum/2
  One_by_Two/1 -> Sum/1
  Switch for rotor alignment/1 -> Switch for Current offset calibration/3
  Vabc_PU/1 -> One_by_Two/1
  Mux2/1 -> Switch for rotor alignment/1
  Mux1/1 -> Switch for Current offset calibration/1, Enable motor control/3
  Constant2/1 -> Mux1/1, Mux1/3, Mux1/2
  Constant3/1 -> Mux2/3, Mux2/2
  Constant4/1 -> Mux2/1
  Enable/1 -> Enable motor control/2
  Mode Selector/2(PositionOffsetEn) -> Switch for rotor alignment/2
  Mode Selector/1(CurrentOffsetEn) -> Switch for Current offset calibration/2
  Enable motor control/1 -> PWM/1
  Switch for Current offset calibration/1 -> Enable motor control/1
  Sum/1 -> Vabc_Sim/1, Switch for rotor alignment/3

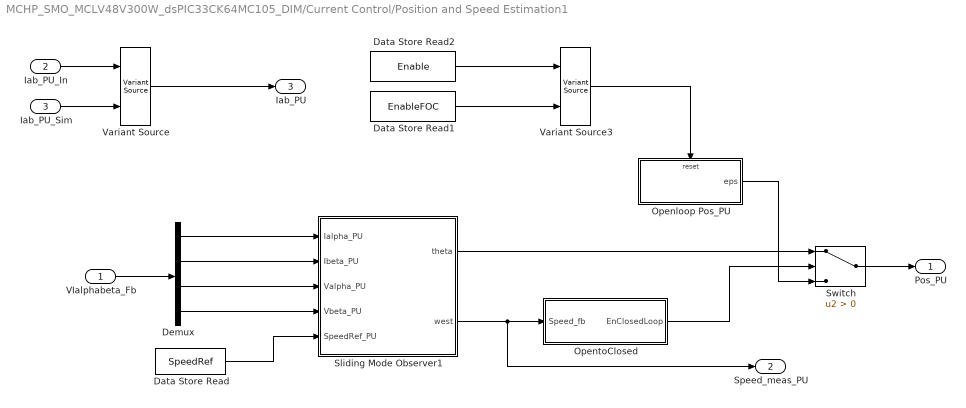
== system MCHP_SMO_MCLV48V300W_dsPIC33CK64MC105_DIM/Current Control/Position and Speed Estimation1 ==
  VIalphabeta_Fb : Inport
  Iab_PU_In : Inport  Port=2
  Iab_PU_Sim : Inport  Port=3
  Data Store Read : DataStoreRead  DataStoreName=SpeedRef  IndexOptions=Index vector (dialog)  Indices=1  OutputSizes=1
  Data Store Read1 : DataStoreRead  DataStoreName=EnableFOC  IndexOptions=Index vector (dialog)  Indices=1  OutputSizes=1
  Data Store Read2 : DataStoreRead  DataStoreName=Enable  IndexOptions=Index vector (dialog)  Indices=1  OutputSizes=1
  Demux : Demux
  Openloop Pos_PU : Subsystem  TreatAsAtomicUnit=on
  OpentoClosed : Subsystem
  Sliding Mode Observer1 : Subsystem
  Switch : Switch  Criteria=u2 > Threshold  SaturateOnIntegerOverflow=off  InputSameDT=off
  Variant Source : VariantSource
  Variant Source3 : VariantSource
  Pos_PU : Outport
  Speed_meas_PU : Outport  Port=2
  Iab_PU : Outport  Port=3
  wires:
  VIalphabeta_Fb/1 -> Demux/1
  Demux/4 -> Sliding Mode Observer1/4(Vbeta_PU)
  Data Store Read/1 -> Sliding Mode Observer1/5(SpeedRef_PU)
  Demux/2 -> Sliding Mode Observer1/2(Ibeta_PU)
  Demux/1 -> Sliding Mode Observer1/1(Ialpha_PU)
  Demux/3 -> Sliding Mode Observer1/3(Valpha_PU)
  Sliding Mode Observer1/2(west) -> Speed_meas_PU/1, OpentoClosed/1(Speed_fb)
  OpentoClosed/1(EnClosedLoop) -> Switch/2
  Sliding Mode Observer1/1(theta) -> Switch/1
  Switch/1 -> Pos_PU/1
  Openloop Pos_PU/1(eps) -> Switch/3
  Variant Source/1 -> Iab_PU/1
  Iab_PU_Sim/1 -> Variant Source/2
  Iab_PU_In/1 -> Variant Source/1
  Data Store Read1/1 -> Variant Source3/2
  Variant Source3/1 -> Openloop Pos_PU/Reset
  Data Store Read2/1 -> Variant Source3/1

== system MCHP_SMO_MCLV48V300W_dsPIC33CK64MC105_DIM/Current Control/Serial Tx ==
  Data : Inport
  Counter Limited : simulink/Sources/Counter Limited  uplimit=3  tsamp=-1
  Data Type Conversion : DataTypeConversion  OutDataTypeStr=uint8  RndMeth=Simplest  SaturateOnIntegerOverflow=off
  Demux : Demux  Outputs=2
  Index Vector : MultiPortSwitch  DataPortOrder=Zero-based contiguous  Inputs=2  DiagnosticForDefault=None  zeroidx=on  OutDataTypeStr=Inherit: Same as first data input  RndMeth=Simplest  SaturateOnIntegerOverflow=off  InputSameDT=off
  UART_TX : Subsystem
  wires:
  Data Type Conversion/1 -> UART_TX/1(Count), Index Vector/1
  Index Vector/1 -> UART_TX/2(Data)
  Demux/1 -> Index Vector/2
  Demux/2 -> Index Vector/3
  Data/1 -> Demux/1
  Counter Limited/1 -> Data Type Conversion/1

== system MCHP_SMO_MCLV48V300W_dsPIC33CK64MC105_DIM/Inverter and Motor/Codegeneration ==
  Duty_Cycles : Inport
  Ground : Ground
  Terminator : Terminator
  Feedbacks_Iab : Outport  VectorParamsAs1DForOutWhenUnconnected=off
  wires:
  Ground/1 -> Feedbacks_Iab/1
  Duty_Cycles/1 -> Terminator/1

== system MCHP_SMO_MCLV48V300W_dsPIC33CK64MC105_DIM/Inverter and Motor/Simulation ==
  Duty_Cycles : Inport
  Inverter : Subsystem
  Load_Profile (Torque) : Subsystem
  Sensor_Measurements : Subsystem
  Surface Mount PMSM : autolibpmsmexterior/Surface Mount PMSM  port_config=Torque  sim_type=Discrete  Ts=Ts  P=pmsm.p  Rs=pmsm.Rs + inverter.R_board  Ldq_=pmsm.Ld  KConstText=Permanent flux linkage constant (lambda_pm):  lambda_pm=pmsm.FluxPM  Ke=159.9771  Kt=1.323  mechanical=[pmsm.J, pmsm.B, 0]  idq0=[0 0]  theta_init=0  omega_init=0  KConst=pmsm.FluxPM  lambda_pm_calc=pmsm.FluxPM  RefBlkName='autolibpmsmexterior/Surface Mount PMSM'  aMode=5  Ldq="[0.0002      0.0002]"
  Terminator : Terminator
  Terminator1 : Terminator
  Feedbacks_Iab : Outport  VectorParamsAs1DForOutWhenUnconnected=off
  wires:
  Duty_Cycles/1 -> Inverter/1(Duty_abc)
  Surface Mount PMSM/2 -> Sensor_Measurements/1(PhaseCurr)  "Iabc"
  Sensor_Measurements/1(Iab_fb) -> Feedbacks_Iab/1
  Load_Profile (Torque)/1(Load_Trq) -> Surface Mount PMSM/1
  Inverter/1(Vabc) -> Surface Mount PMSM/2
  Surface Mount PMSM/3 -> Terminator/1
  Surface Mount PMSM/1 -> Terminator1/1

== system MCHP_SMO_MCLV48V300W_dsPIC33CK64MC105_DIM/Speed Control/Enable Switch ==
  Codegen : Subsystem  VariantControl=(codegen)
  Sim : Subsystem  VariantControl=(sim)

== system MCHP_SMO_MCLV48V300W_dsPIC33CK64MC105_DIM/Speed Control/PI_Controller_Speed ==
  N_ref : Inport
  N_fb : Inport  Port=2
  AND : Logic  IconShape=distinctive  AllPortsSameDT=off  OutDataTypeStr=boolean
  Data Store Read1 : DataStoreRead  DataStoreName=EnableClosedLoop  IndexOptions=Index vector (dialog)  Indices=1  OutputSizes=1
  Data Store Read2 : DataStoreRead  DataStoreName=Enable  IndexOptions=Index vector (dialog)  Indices=1  OutputSizes=1
  Discrete PI Controller with anti-windup & reset : slpidlib/PID Controller  Controller=PI  Form=Parallel  TimeDomain=Discrete-time  UseExternalTs=off  SampleTime=-1  IntegratorMethod=Forward Euler  FilterMethod=Forward Euler  ControllerParametersSource=external  P=1  I=1  UseKiTs=on  D=0  N=100  UseFilter=on  TunerSelectOption=Transfer Function Based (PID Tuner App)  InitialConditionSource=external  InitialConditionForIntegrator=0  InitialConditionForFilter=0  DifferentiatorICPrevScaledInput=0  ExternalReset=level  TrackingMode=off  Kt=1  LimitOutput=on  SatLimitsSource=internal  UpperSaturationLimit=1  LowerSaturationLimit=-1  LinearizeAsGain=on  AntiWindupMode=clamping  Kb=1  LimitIntegrator=off  UpperIntegratorSaturationLimit=inf  LowerIntegratorSaturationLimit=-inf  RndMeth=Simplest  POutMin=[]  POutMax=[]  IOutMin=[]  IOutMax=[]  DOutMin=[]  DOutMax=[]  NOutMin=[]  NOutMax=[]  SumOutMin=[]  SumOutMax=[]  SaturationOutDataTypeStr=Inherit: Inherit via back propagation  SaturationOutMin=[]  SaturationOutMax=[]  PParamMin=[]  PParamMax=[]  IParamMin=[]  IParamMax=[]  DParamMin=[]  DParamMax=[]  NParamMin=[]  NParamMax=[]  KbParamMin=[]  KbParamMax=[]  KtParamMin=[]  KtParamMax=[]  KbOutMin=[]  KbOutMax=[]  KtOutMin=[]  KtOutMax=[]  IntegratorOutMin=[]  IntegratorOutMax=[]  FilterOutMin=[]  FilterOutMax=[]  SumI1OutMin=[]  SumI1OutMax=[]  SumI2OutMin=[]  SumI2OutMax=[]  SumI3OutMin=[]  SumI3OutMax=[]  SumI4OutMin=[]  SumI4OutMax=[]  SumDOutMin=[]  SumDOutMax=[]  DifferentiatorOutMin=[]  DifferentiatorOutMax=[]  FilterDiffOutCoefMin=[]  FilterDiffOutCoefMax=[]  ReciprocalOutMin=[]  ReciprocalOutMax=[]  SumDenOutMin=[]  SumDenOutMax=[]  SumNumOutMin=[]  SumNumOutMax=[]  DivideOutMin=[]  DivideOutMax=[]  UdiffTsProdOutMin=[]  UdiffTsProdOutMax=[]  NTsProdOutMin=[]  NTsProdOutMax=[]  UintegralTsProdOutMin=[]  UintegralTsProdOutMax=[]  UngainTsProdOutMin=[]  UngainTsProdOutMax=[]  ClampingZeroOutDataTypeStr=Inherit: Inherit via back propagation  ClampingZeroOutMin=[]  ClampingZeroOutMax=[]  FilterDenConstantOutDataTypeStr=Inherit: Inherit via back propagation  FilterDenConstantOutMin=[]  FilterDenConstantOutMax=[]  PCopyOutDataTypeStr=Inherit: Inherit via back propagation  PCopyOutMin=[]  PCopyOutMax=[]  NCopyOutDataTypeStr=Inherit: Inherit via back propagation  NCopyOutMin=[]  NCopyOutMax=[]  IntegratorContinuousStateAttributes=''  IntegratorStateMustResolveToSignalObject=off  IntegratorRTWStateStorageClass=Auto  FilterContinuousStateAttributes=''  FilterStateMustResolveToSignalObject=off  FilterRTWStateStorageClass=Auto  ParallelPVariant=ExternalParameters  IdealPVariant=Disabled  IVariant=ExternalParameters  DVariant=Disabled  IntegratorVariant=Discrete  SatVariant=Enabled  AWVariant=DiscClampingParallel  PCopyVariant=Disabled  TRVariant=Disabled  FdbkBlocksVariant=Forward  IdealPFdbkVariant=Disabled  SatFdbkVariant=Disabled  DerivativeFilterVariant=Disabled  NVariant=Disabled  NCopyVariant=Disabled_SignalSpec  FilterICVariant=Disabled  IntegratorICVariant=ExternalICs  ExternalResetVariant=ExternalReset  TRSumVariant=Passthrough  SumFdbkVariant=Disabled  SumVariant=Sum_PI  TsampFilterVariant=InternalTs  TsampNgainVariant=Passthrough  TsampIntegralVariant=Passthrough  ExternalSaturationOutDataTypeStr=Inherit: Same as second input
  Ki1 : Constant  Value=(PI_params.Ki_speed*Ts_speed)  OutDataTypeStr=dataType  SampleTime=-1
  Ki2 : Constant  Value=0  OutDataTypeStr=dataType  SampleTime=-1
  Kp1 : Constant  Value=PI_params.Kp_speed  OutDataTypeStr=dataType  SampleTime=-1
  Logical Operator : Logic  Operator=NOT  IconShape=distinctive  AllPortsSameDT=off  OutDataTypeStr=boolean
  Sum : Sum  Inputs=|+-  OutDataTypeStr=Inherit: Same as first input
  Zero_Cancellation : mcbcontrolslib/IIR Filter  VariantControl=Low Pass Filter  VariantSelect=Low-pass  Filter_constant=0.001*(Ts_speed/Ts)  advancedSettings=off  Ts=50e-6  cutOff_freq=98.4464
  Iq_ref : Outport  VectorParamsAs1DForOutWhenUnconnected=off
  wires:
  Discrete PI Controller with anti-windup & reset/1 -> Iq_ref/1
  Ki1/1 -> Discrete PI Controller with anti-windup & reset/3
  Kp1/1 -> Discrete PI Controller with anti-windup & reset/2
  N_fb/1 -> Sum/2
  N_ref/1 -> Zero_Cancellation/1
  Sum/1 -> Discrete PI Controller with anti-windup & reset/1
  Logical Operator/1 -> Discrete PI Controller with anti-windup & reset/4
  Ki2/1 -> Discrete PI Controller with anti-windup & reset/5
  Zero_Cancellation/1 -> Sum/1
  AND/1 -> Logical Operator/1
  Data Store Read1/1 -> AND/1
  Data Store Read2/1 -> AND/2

== system MCHP_SMO_MCLV48V300W_dsPIC33CK64MC105_DIM/Speed Control/Speed_Ref_Selector ==
  Speed_Ref_In : Inport
  Constant : Constant  Value=0  OutDataTypeStr=dataType  SampleTime=Ts_speed
  Data Store Read1 : DataStoreRead  DataStoreName=EnableFOC  IndexOptions=Index vector (dialog)  Indices=1  OutputSizes=1
  Switch : Switch  Criteria=u2 > Threshold  Threshold=0.5  SaturateOnIntegerOverflow=off  InputSameDT=off
  Speed_Ref_PU : Outport
  wires:
  Switch/1 -> Speed_Ref_PU/1
  Constant/1 -> Switch/3
  Speed_Ref_In/1 -> Switch/1
  Data Store Read1/1 -> Switch/2

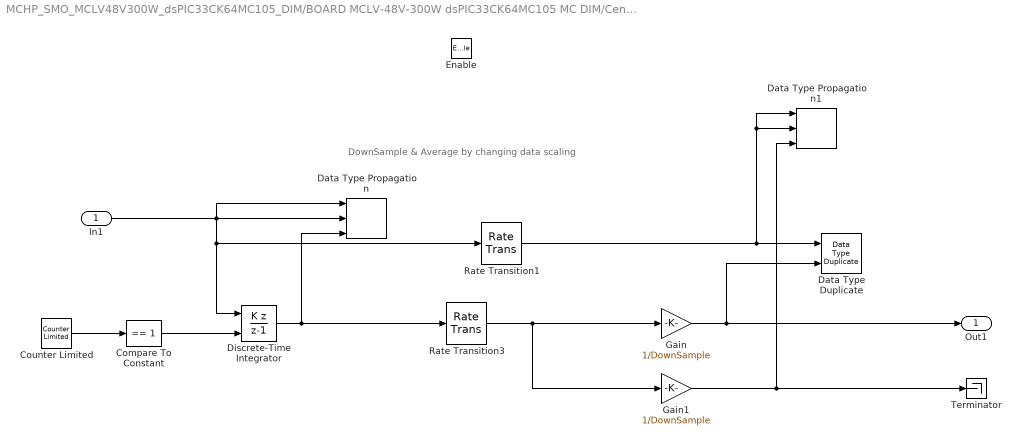
== system MCHP_SMO_MCLV48V300W_dsPIC33CK64MC105_DIM/BOARD MCLV-48V-300W dsPIC33CK64MC105 MC DIM/Center & sign reversal/Downsample Averaged 2000 samples remove bias ==
  note: DownSample & Average by changing data scaling
  In1 : Inport
  Enable : EnablePort
  Compare To Constant : simulink/Logic and Bit Operations/Compare To Constant  relop===  const=1  OutDataTypeStr=boolean
  Counter Limited : simulink/Sources/Counter Limited  uplimit=DownSample-1  tsamp=-1
  Data Type Duplicate : DataTypeDuplicate
  Data Type Propagation : simulink/Signal Attributes/Data Type Propagation  PropDataType=fixdt(1, 16)  IfRefDouble=double  IfRefSingle=single  IsSigned=IsSigned1 or IsSigned2  NumBitsBase=NumBits1+NumBits2  NumBitsMult=1  NumBitsAdd=0  NumBitsAllowFinal=1:128  PropScaling=2^-10  ValuesUsedBestPrec=[5 -7]  SlopeBase=Slope1  SlopeMult=1  SlopeAdd=0  BiasBase=Bias1  BiasMult=1  BiasAdd=0
  Data Type Propagation1 : simulink/Signal Attributes/Data Type Propagation  PropDataType=fixdt(1, 16)  IfRefDouble=double  IfRefSingle=single  IsSigned=IsSigned1 or IsSigned2  NumBitsBase=NumBits1+NumBits2  NumBitsMult=1  NumBitsAdd=0  NumBitsAllowFinal=1:128  PropScaling=2^-10  ValuesUsedBestPrec=[5 -7]  SlopeBase=PosRange1  SlopeMult=1  SlopeAdd=0  BiasBase=Bias1  BiasMult=1  BiasAdd=0
  Discrete-Time Integrator : DiscreteIntegrator  IntegratorMethod=Accumulation: Backward Euler  gainval=1  ExternalReset=sampled level  SampleTime=-1  OutDataTypeStr=Inherit: Inherit via back propagation  ICPrevOutput=DiscIntNeverNeededParam  ICPrevScaledInput=DiscIntNeverNeededParam
  Gain : Gain  Gain=1/DownSample  OutDataTypeStr=Inherit: Inherit via back propagation  RndMeth=Round
  Gain1 : Gain  Gain=1/DownSample  OutDataTypeStr=Inherit: Inherit via back propagation
  Rate Transition1 : RateTransition  OutPortSampleTimeOpt=Multiple of input port sample time  OutPortSampleTimeMultiple=DownSample  OutPortSampleTime=DownSample
  Rate Transition3 : RateTransition  OutPortSampleTimeOpt=Multiple of input port sample time  OutPortSampleTimeMultiple=DownSample  OutPortSampleTime=DownSample
  Terminator : Terminator
  Out1 : Outport  VectorParamsAs1DForOutWhenUnconnected=off
  wires:
  Gain1/1 -> Data Type Propagation1/3, Terminator/1
  Rate Transition1/1 -> Data Type Duplicate/1, Data Type Propagation1/1, Data Type Propagation1/2
  Gain/1 -> Out1/1, Data Type Duplicate/2
  Counter Limited/1 -> Compare To Constant/1
  Discrete-Time Integrator/1 -> Rate Transition3/1, Data Type Propagation/3
  Compare To Constant/1 -> Discrete-Time Integrator/2
  In1/1 -> Data Type Propagation/1, Data Type Propagation/2, Discrete-Time Integrator/1, Rate Transition1/1
  Rate Transition3/1 -> Gain/1, Gain1/1

== system MCHP_SMO_MCLV48V300W_dsPIC33CK64MC105_DIM/BOARD MCLV-48V-300W dsPIC33CK64MC105 MC DIM/Timing Analysis/Downsample Averaged2 ==
  note: DownSample & Average by changing data scaling
  In1 : Inport
  Compare To Constant : simulink/Logic and Bit Operations/Compare To Constant  relop===  const=1  OutDataTypeStr=boolean
  Counter Limited : simulink/Sources/Counter Limited  uplimit=DownSample-1  tsamp=-1
  Data Type Duplicate : DataTypeDuplicate
  Data Type Propagation : simulink/Signal Attributes/Data Type Propagation  PropDataType=fixdt(1, 16)  IfRefDouble=double  IfRefSingle=single  IsSigned=IsSigned1 or IsSigned2  NumBitsBase=NumBits1+NumBits2  NumBitsMult=1  NumBitsAdd=0  NumBitsAllowFinal=1:128  PropScaling=2^-10  ValuesUsedBestPrec=[5 -7]  SlopeBase=Slope1  SlopeMult=1  SlopeAdd=0  BiasBase=Bias1  BiasMult=1  BiasAdd=0
  Data Type Propagation1 : simulink/Signal Attributes/Data Type Propagation  PropDataType=fixdt(1, 16)  IfRefDouble=double  IfRefSingle=single  IsSigned=IsSigned1 or IsSigned2  NumBitsBase=NumBits1+NumBits2  NumBitsMult=1  NumBitsAdd=0  NumBitsAllowFinal=1:128  PropScaling=2^-10  ValuesUsedBestPrec=[5 -7]  SlopeBase=PosRange1  SlopeMult=1  SlopeAdd=0  BiasBase=Bias1  BiasMult=1  BiasAdd=0
  Discrete-Time Integrator : DiscreteIntegrator  IntegratorMethod=Accumulation: Backward Euler  gainval=1  ExternalReset=sampled level  SampleTime=-1  OutDataTypeStr=Inherit: Inherit via back propagation  ICPrevOutput=DiscIntNeverNeededParam  ICPrevScaledInput=DiscIntNeverNeededParam
  Gain : Gain  Gain=1/DownSample  OutDataTypeStr=Inherit: Inherit via back propagation
  Gain1 : Gain  Gain=1/DownSample  OutDataTypeStr=Inherit: Inherit via back propagation
  Rate Transition1 : RateTransition  Deterministic=off  OutPortSampleTime=[InputSampleTime * DownSample]
  Rate Transition3 : RateTransition  OutPortSampleTime=[InputSampleTime * DownSample]
  Terminator : Terminator
  Out1 : Outport  VectorParamsAs1DForOutWhenUnconnected=off
  wires:
  Rate Transition3/1 -> Gain1/1, Gain/1
  In1/1 -> Discrete-Time Integrator/1, Rate Transition1/1, Data Type Propagation/2, Data Type Propagation/1
  Compare To Constant/1 -> Discrete-Time Integrator/2
  Discrete-Time Integrator/1 -> Data Type Propagation/3, Rate Transition3/1
  Counter Limited/1 -> Compare To Constant/1
  Gain/1 -> Data Type Duplicate/2, Out1/1
  Rate Transition1/1 -> Data Type Propagation1/2, Data Type Propagation1/1, Data Type Duplicate/1
  Gain1/1 -> Data Type Propagation1/3, Terminator/1

== system MCHP_SMO_MCLV48V300W_dsPIC33CK64MC105_DIM/Current Control/Closed Loop Control1/Current_Controllers ==
  Id : Inport
  Iq : Inport  Port=2
  Idq_ref_PU : Inport  Port=3
  DQ Limiter : mcbcontrolslib/DQ Limiter  satMethodInputType=Specify via dialog  satMethodSelected=D-Q equivalence  satLimitInputType=Specify via dialog  Vmax=0.95
  Demux : Demux  Outputs=2
  Mux : Mux
  PI_Controller_Id : Subsystem
  PI_Controller_Iq : Subsystem
  Terminator : Terminator
  Terminator1 : Terminator
  Vd_ref : Outport  VectorParamsAs1DForOutWhenUnconnected=off
  Vq_ref : Outport  Port=2  VectorParamsAs1DForOutWhenUnconnected=off
  wires:
  Iq/1 -> Mux/4, PI_Controller_Iq/2(I_fb)  "Iq_fb"
  Id/1 -> Mux/2, PI_Controller_Id/2(I_fb)  "Id_fb"
  Demux/1 -> Mux/1, PI_Controller_Id/1(I_ref)  "Id_Ref"
  Demux/2 -> Mux/3, PI_Controller_Iq/1(I_ref)  "Iq_Ref"
  Idq_ref_PU/1 -> Demux/1
  PI_Controller_Id/1(V_ref) -> DQ Limiter/1
  PI_Controller_Iq/1(V_ref) -> DQ Limiter/2
  DQ Limiter/1 -> Vd_ref/1
  DQ Limiter/2 -> Vq_ref/1
  DQ Limiter/3 -> Terminator/1
  Mux/1 -> Terminator1/1

== system MCHP_SMO_MCLV48V300W_dsPIC33CK64MC105_DIM/Current Control/Output Scaling/Mode Selector ==
  Delay : Delay  DelayLength=1
  NOT : Logic  Operator=NOT  IconShape=distinctive  AllPortsSameDT=off  OutDataTypeStr=boolean
  Subsystem1 : Subsystem
  Up Counter : Subsystem
  CurrentOffsetEn : Outport
  PositionOffsetEn : Outport  Port=2
  wires:
  Subsystem1/2(PositionOffset) -> PositionOffsetEn/1
  Up Counter/1(Count) -> Subsystem1/1(Count)
  Subsystem1/1(Current Offset) -> CurrentOffsetEn/1
  Delay/1 -> NOT/1
  NOT/1 -> Up Counter/Enable
  Subsystem1/3(EnableFOC) -> Delay/1
